simulink model "Callback"  (R2024a)
settings: Solver=FixedStepAuto  StartTime=0.0  StopTime=10  FixedStep=TensionSampleTime  RelTol=1e-3
model workspace (MAT data in the model file):
  TensionSampleTime = 0.001
libraries: sldrtlib x1
settings Model: SimulationMode=accelerator  Creator=17739  LastModifiedBy=17739
settings SolverCC: PositivePriorityOrder=on
settings OptimizationCC: BlockReduction=off  DefaultParameterBehavior=Inlined  OptimizeBlockIOStorage=off  EnhancedBackFolding=on  PassReuseOutputArgsThreshold=0  OptimizeBlockOrder=speed  DifferentSizesBufferReuse=on
settings DebuggingCC: TasksWithSamePriorityMsg=none  ParameterTunabilityLossMsg=error
settings HardwareCC: ProdBitPerLong=64  ProdHWDeviceType=Intel->x86-64 (Linux 64)
settings SFSimCC: MATLABDynamicMemAlloc=off
settings RTWCC: Description=Simulink Desktop Real-Time  SystemTargetFile=sldrt.tlc  TemplateMakefile=sldrt.tmf  Toolchain=Simulink Real-Time Toolchain  BuildConfiguration=Faster Runs  TargetLang=C++  RTWCompilerOptimization=on  GPUComputeCapability=3.5
settings CodeAppCC: ForceParamTrailComments=on  MaxIdLength=95  OperatorAnnotations=on
settings SimulinkDesktopRealTimeCC: TargetLibSuffix=_sldrt.a  TargetPreCompLibLocation=C:\MATLAB\R2024a\toolbox\sldrt\lib\win64  TargetLangStandard=C++03 (ISO)

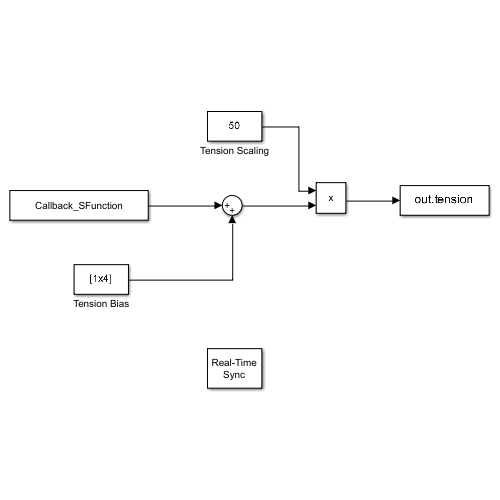
[thumbnail: Simulink's stored preview of the top-level diagram]
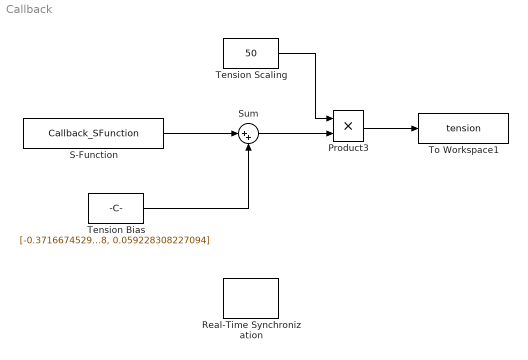
== system Callback ==
  Product3 : Product
  Real-Time Synchronization : sldrtlib/Real-Time Synchronization  SampleTime=TensionSampleTime  MaxMissedTicks=inf  ShowMissedTicks=off  YieldWhenWaiting=off
  S-Function : S-Function  FunctionName=Callback_SFunction  SFunctionDeploymentMode=off  EnableBusSupport=off
  Sum : Sum  Inputs=|++
  Tension Bias : Constant  Value=[-0.371667452961505, -0.378134600005407, -0.142699350266888, 0.059228308227094]
  Tension Scaling : Constant  Value=50
  To Workspace1 : ToWorkspace  VariableName=tension  SampleTime=-1
  wires:
  Tension Bias/1 -> Sum/2
  Product3/1 -> To Workspace1/1
  Tension Scaling/1 -> Product3/1
  S-Function/1 -> Sum/1
  Sum/1 -> Product3/2
